simulink model "dds_test"  (Simulink 7.4)
settings: Solver=ode45  StartTime=0.0  StopTime=1000  RelTol=1e-3
libraries: xbsIndex_r4 x23, simulink x2
(part 4 of 5)

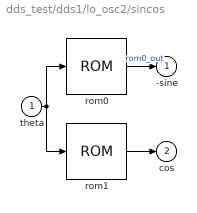
== system dds_test/dds1/lo_osc2/sincos ==
  theta : Inport
  rom0 : xbsIndex_r4/ROM  depth=2048  initVector=[-0 -0.00306795676296598 -0.00613588464915448 -0.00920375478205982 -0.0122715382857199 -0.0153392062849881 -0.0184067299058048 -0.0214740802754695 -0.0245412285229123 -0.0276081457789657 -0.0306748031766366 -0.0337411718513776 -0.0368072229413588 -0.0398729275877398 -0.0429382569349408 -0.0460031821309146 -0.049067674327418 -0.0521317046802833 -0.0551952443496899 -0.0582582645004358 -0.0613207363022086 -0.0643826309298575 -0.0674439195636641 -0.0705045733896139 -0.0735645635996674 -0.0766238613920315 -0.0796824379714301 -0.0827402645493757 -0.0857973123444399 -0.0888535525825246 -0.0919089564971327 -0.094963495329639 -0.0980171403295606 -0.101069862754828 -0.104121633872055 -0.107172424956809 -0.110222207293883 -0.113270952177564 -0.116318630911905 -0.119365214810991 -0.122410675199216 -0.125454983411546 -0.128498110793793 -0.131540028702883 -0.134580708507126 -0.137620121586486 -0.140658239332849 -0.143695033150294 -0.146730474455362 -0.149764534677322 -0.152797185258443 -0.155828397654265 -0.158858143333861 -0.161886393780112 -0.16491312048997 -0.167938294974731 -0.170961888760301 -0.173983873387464 -0.177004220412149 -0.1800229014057 -0.183039887955141 -0.186055151663447 -0.189068664149806 -0.192080397049892 -0.195090322016128 -0.198098410717954 -0.201104634842092 -0.204108966092817 -0.207111376192219 -0.21011183688047 -0.213110319916091 -0.21610679707622 -0.21910124015687 -0.222093620973204 -0.225083911359793 -0.228072083170886 -0.231058108280671 -0.234041958583543 -0.237023605994367 -0.240003022448741 -0.242980179903264 -0.245955050335795 -0.24892760574572 -0.251897818154217 -0.254865659604515 -0.257831102162159 -0.260794117915276 -0.263754678974831 -0.266712757474898 -0.269668325572915 -0.272621355449949 -0.275571819310958 -0.278519689385053 -0.281464937925758 -0.284407537211272 -0.28734745954473 -0.290284677254462 -0.293219162694259 -0.296150888243624 -0.29907982630804 -0.302005949319228 -0.304929229735402 -0.307849640041535 -0.310767152749611 -0.313681740398892 -0.316593375556166 -0.319502030816016 -0.32240767880107 -0.325310292162263 -0.328209843579092 -0.331106305759876 -0.333999651442009 -0.33688985339222 -0.339776884406827 -0.342660717311994 -0.345541324963989 -0.348418680249435 -0.351292756085567 -0.35416352542049 -0.35703096123343 -0.359895036534988 -0.362755724367397 -0.365612997804774 -0.368466829953372 -0.371317193951837 -0.374164062971458 -0.377007410216418 -0.379847208924051 -0.38268343236509 -0.385516053843919 -0.388345046698826 -0.391170384302254 -0.393992040061048 -0.39680998741671 -0.399624199845647 -0.402434650859418 -0.40524131400499 -0.408044162864979 -0.410843171057904 -0.413638312238435 -0.416429560097637 -0.419216888363224 -0.4220002707998 -0.424779681209109 -0.427555093430282 -0.430326481340083 -0.433093818853152 -0.435857079922255 -0.438616238538528 -0.441371268731717 -0.444122144570429 -0.446868840162374 -0.449611329654607 -0.452349587233771 -0.455083587126344 -0.457813303598877 -0.46053871095824 -0.46325978355186 -0.465976495767966 -0.468688822035828 -0.471396736825998 -0.47410021465055 -0.476799230063322 -0.479493757660153 -0.482183772079123 -0.484869248000791 -0.487550160148436 -0.490226483288291 -0.492898192229784 -0.495565261825773 -0.498227666972782 -0.500885382611241 -0.503538383725718 -0.506186645345155 -0.508830142543107 -0.51146885043797 -0.514102744193222 -0.51673179901765 -0.51935599016559 -0.521975292937154 -0.524589682678469 -0.527199134781901 -0.529803624686295 -0.532403127877198 -0.534997619887097 -0.537587076295645 -0.540171472729893 -0.542750784864516 -0.545324988422046 -0.5478940591731 -0.550457972936605 -0.553016705580027 -0.555570233019602 -0.558118531220556 -0.560661576197336 -0.563199344013834 -0.565731810783613 -0.568258952670131 -0.570780745886967 -0.573297166698042 -0.575808191417845 -0.578313796411656 -0.580813958095765 -0.583308652937698 -0.585797857456439 -0.588281548222645 -0.590759701858874 -0.5932322950398 -0.595699304492433 -0.598160706996342 -0.600616479383869 ...(+33739 chars)]  distributed_mem=Block RAM  rst=off  init_reg=0  en=off  latency=2  arith_type="Signed  (2's comp)"  n_bits=8  bin_pt=7  dbl_ovrd=off  optimize=Area  use_rpm=on  block_type=sprom
      settings: block_version=11.4
  rom1 : xbsIndex_r4/ROM  depth=2048  initVector=[1 0.999995293809576 0.999981175282601 0.999957644551964 0.999924701839145 0.999882347454213 0.999830581795823 0.999769405351215 0.999698818696204 0.999618822495179 0.999529417501093 0.999430604555462 0.99932238458835 0.999204758618364 0.999077727752645 0.998941293186857 0.998795456205172 0.998640218180265 0.998475580573295 0.998301544933893 0.998118112900149 0.997925286198596 0.997723066644192 0.997511456140303 0.99729045667869 0.997060070339483 0.996820299291166 0.996571145790555 0.996312612182778 0.996044700901252 0.99576741446766 0.995480755491927 0.995184726672197 0.994879330794806 0.994564570734255 0.994240449453188 0.993906970002356 0.993564135520595 0.993211949234795 0.992850414459865 0.99247953459871 0.992099313142192 0.9917097536691 0.991310859846115 0.99090263542778 0.990485084256457 0.990058210262297 0.989622017463201 0.989176509964781 0.988721691960324 0.988257567730749 0.987784141644572 0.987301418157858 0.986809401814186 0.986308097244599 0.985797509167567 0.985277642388941 0.984748501801904 0.984210092386929 0.98366241921173 0.983105487431216 0.982539302287441 0.981963869109555 0.981379193313755 0.98078528040323 0.980182135968117 0.979569765685441 0.978948175319062 0.978317370719628 0.97767735782451 0.977028142657754 0.976369731330021 0.975702130038529 0.975025345066994 0.974339382785576 0.973644249650812 0.97293995220556 0.972226497078936 0.971503890986252 0.97077214072895 0.970031253194544 0.969281235356549 0.968522094274417 0.967753837093476 0.966976471044852 0.966190003445413 0.965394441697689 0.964589793289813 0.96377606579544 0.962953266873684 0.962121404269042 0.961280485811321 0.960430519415566 0.959571513081985 0.958703474895872 0.957826413027533 0.956940335732209 0.956045251349996 0.955141168305771 0.954228095109106 0.953306040354194 0.952375012719766 0.951435020969008 0.950486073949482 0.949528180593037 0.94856134991573 0.947585591017741 0.946600913083284 0.945607325380521 0.94460483726148 0.94359345816196 0.942573197601447 0.941544065183021 0.940506070593268 0.93945922360219 0.938403534063108 0.937339011912575 0.936265667170278 0.935183509938948 0.934092550404259 0.932992798834739 0.931884265581668 0.930766961078984 0.929640895843181 0.928506080473216 0.927362525650401 0.926210242138311 0.925049240782678 0.923879532511287 0.922701128333879 0.921514039342042 0.920318276709111 0.919113851690058 0.91790077562139 0.916679059921043 0.915448716088268 0.914209755703531 0.912962190428398 0.91170603200543 0.910441292258067 0.909167983090522 0.907886116487666 0.906595704514915 0.905296759318119 0.903989293123443 0.902673318237259 0.901348847046022 0.90001589201616 0.898674465693954 0.897324580705418 0.895966249756185 0.894599485631383 0.893224301195515 0.891840709392343 0.890448723244758 0.889048355854665 0.887639620402854 0.886222530148881 0.884797098430938 0.883363338665732 0.881921264348355 0.880470889052161 0.879012226428634 0.877545290207261 0.876070094195407 0.874586652278176 0.87309497841829 0.871595086655951 0.870086991108711 0.868570705971341 0.867046245515693 0.865513624090569 0.863972856121587 0.862423956111041 0.860866938637767 0.859301818357008 0.857728610000272 0.856147328375194 0.854557988365401 0.852960604930364 0.851355193105265 0.849741768000853 0.848120344803297 0.846490938774052 0.844853565249707 0.843208239641845 0.841554977436898 0.839893794196 0.838224705554838 0.836547727223512 0.83486287498638 0.833170164701913 0.831469612302545 0.829761233794523 0.828045045257756 0.826321062845664 0.824589302785025 0.822849781375826 0.821102514991105 0.819347520076797 0.817584813151584 0.815814410806734 0.814036329705948 0.812250586585204 0.810457198252595 0.808656181588175 0.806847553543799 0.805031331142964 0.803207531480645 0.80137617172314 0.799537269107905 0.797690840943391 0.795836904608884 0.793975477554337 0.792106577300212 0.79023022143731 0.788346427626606 0.786455213599086 0.784556597155575 0.782650596166576 0.780737228572094 0.778816512381476 0.776888465673232 0.774953106594874 ...(+33759 chars)]  distributed_mem=Block RAM  rst=off  init_reg=0  en=off  latency=2  arith_type="Signed  (2's comp)"  n_bits=8  bin_pt=7  dbl_ovrd=off  optimize=Area  use_rpm=on  block_type=sprom
      settings: block_version=11.4
  -sine : Outport
  cos : Outport  Port=2
  wires:
  theta/1 -> rom1/1, rom0/1
  rom1/1 -> cos/1
  rom0/1 -> -sine/1  "rom0_out"
